simulink model "test_stepper_vector_space"  (R2020b)
settings: Solver=VariableStepAuto  StartTime=0.0  StopTime=10.0  RelTol=1e-3
undefined symbols (not defined in the file): const, controller, stepper
settings Model: Creator=Utente  LastModifiedBy=Utente

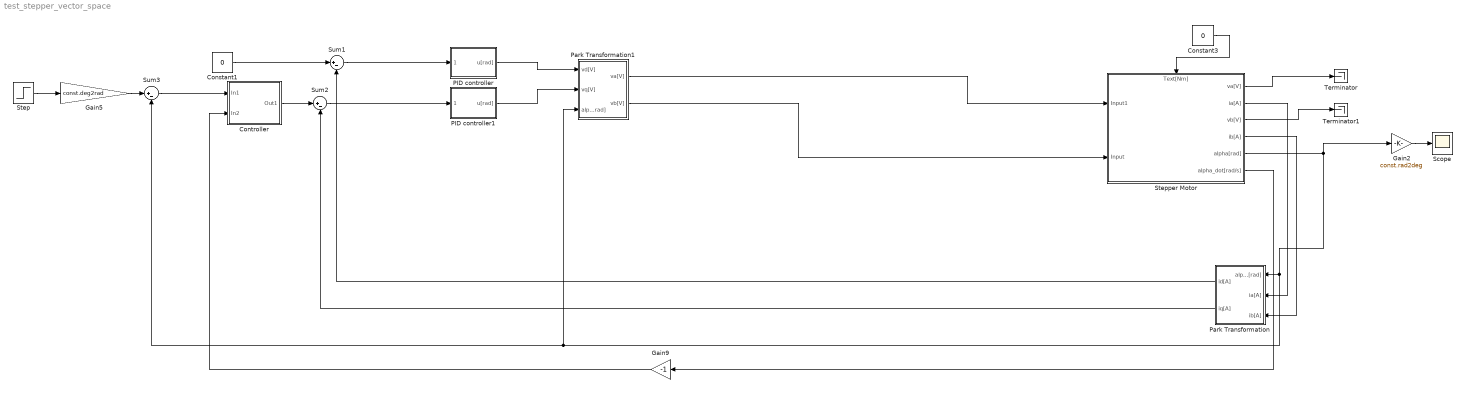
== system test_stepper_vector_space ==
  Constant1 : Constant  Value=0
  Constant3 : Constant  Value=0
  Controller : Subsystem
  Gain2 : Gain  Gain=const.rad2deg
  Gain5 : Gain  Gain=const.deg2rad
  Gain9 : Gain  Gain=-1
  PID controller : Subsystem
  PID controller1 : Subsystem
  Park Transformation : Subsystem
  Park Transformation1 : Subsystem
  Scope : Scope
  Step : Step  Time=0.1  After=30  SampleTime=0
  Stepper Motor : Subsystem
      settings: PortSchema="{\"entries\":[{\"content\":{\"sides\":[{\"content\":{\"connectorIds\":[\"In1\",\"In2\"]},\"type\":\"ConnectorPlacement.EquallySpacedRectSide\",\"uuid\":\"73295f7e-2188-4526-b3fe-31d6eab8afcb\"},{\"content\":{\"connectorIds\":[\"Out1\",\"Out2\",\"Out3\",\"Out4\",\"Out5\",\"Out6\"],\"side\":\"RIGHT\"},\"type\":\"ConnectorPlacement.EquallySpacedRectSide\",\"uuid\":\"77dcaa74-ce65-4a13-97c5-e825e2410182\"},{\"content\":{\"connectorIds\":[\"In3\"],\"side\":\"TOP\"},\"type\":\"ConnectorPlacement.EquallySpacedRectSide\",\"uuid\":\"bac6b674-d00a-4490-8f08-a2567c8e6873\"},{\"content\":{\"connectorIds\":[],\"side\":\"HIDDEN\"},\"type\":\"ConnectorPlacement.EquallySpacedRectSide\",\"uuid\":\"66c41dc0-366a-490c-a787-062f795e6cc7\"}]},\"type\":\"ConnectorPlacement.EquallySpacedConnector\",\"uuid\":\"3c22aa21-f88d-4b07-855c-a69922a8689b\"}],\"packageUris\":[\"http://schema.mathworks.com/mf0/Connector/R2020b\"],\"version\":\"1.0\"}"
  Sum1 : Sum  Inputs=|+-
  Sum2 : Sum  Inputs=|+-
  Sum3 : Sum  Inputs=|+-
  Terminator : Terminator
  Terminator1 : Terminator
  wires:
  Sum2/1 -> PID controller1/1(e[deg])
  Gain5/1 -> Sum3/1
  Sum1/1 -> PID controller/1(e[deg])
  Step/1 -> Gain5/1
  Constant3/1 -> Stepper Motor/3(Text[Nm])
  Park Transformation/2(iq[A]) -> Sum2/2
  Park Transformation/1(id[A]) -> Sum1/2
  Constant1/1 -> Sum1/1
  Stepper Motor/5(alpha[rad]) -> Gain2/1, Park Transformation1/3(alpha[rad]), Sum3/2, Park Transformation/1(alpha[rad])
  Stepper Motor/2(ia[A]) -> Park Transformation/2(ia[A])
  Stepper Motor/4(ib[A]) -> Park Transformation/3(ib[A])
  Stepper Motor/6(alpha_dot[rad/s]) -> Gain9/1
  Sum3/1 -> Controller/1(In1)
  Gain9/1 -> Controller/2(In2)
  Controller/1(Out1) -> Sum2/1
  PID controller/1(u[rad]) -> Park Transformation1/1(vd[V])
  PID controller1/1(u[rad]) -> Park Transformation1/2(vq[V])
  Gain2/1 -> Scope/1
  Stepper Motor/1(va[V]) -> Terminator/1
  Stepper Motor/3(vb[V]) -> Terminator1/1
  Park Transformation1/1(va[V]) -> Stepper Motor/1(Input1)
  Park Transformation1/2(vb[V]) -> Stepper Motor/2(Input)

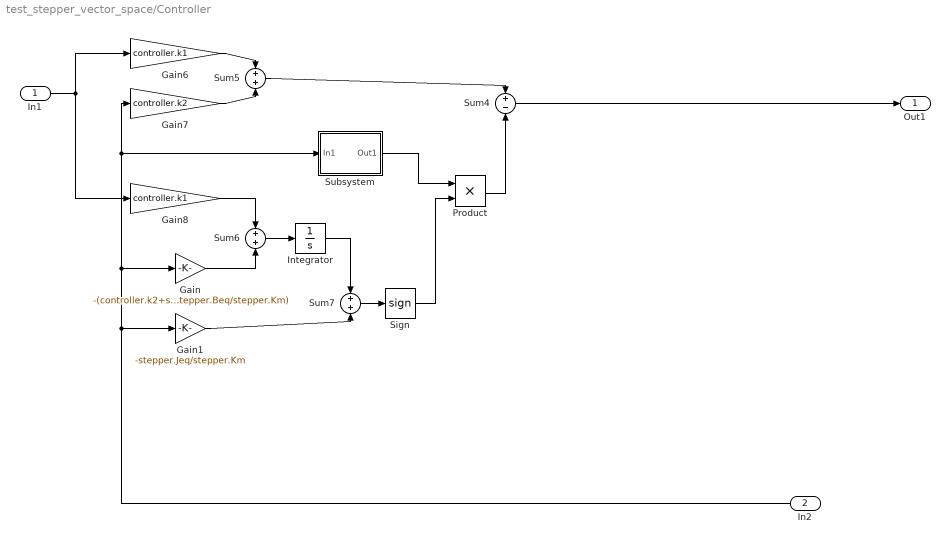
== system test_stepper_vector_space/Controller ==
  In1 : Inport
  In2 : Inport  Port=2
  Gain : Gain  Gain=-(controller.k2+stepper.Beq/stepper.Km)
  Gain1 : Gain  Gain=-stepper.Jeq/stepper.Km
  Gain6 : Gain  Gain=controller.k1
  Gain7 : Gain  Gain=controller.k2
  Gain8 : Gain  Gain=controller.k1
  Integrator : Integrator
  Product : Product
  Sign : Signum  ZeroCross=off
  Subsystem : Subsystem
  Sum4 : Sum  Inputs=+-
  Sum5 : Sum
  Sum6 : Sum
  Sum7 : Sum
  Out1 : Outport
  wires:
  In2/1 -> Subsystem/1(In1), Gain7/1, Gain/1, Gain1/1
  Sum5/1 -> Sum4/1
  Sum7/1 -> Sign/1
  Integrator/1 -> Sum7/1
  Gain1/1 -> Sum7/2
  Gain/1 -> Sum6/2
  Sum4/1 -> Out1/1
  In1/1 -> Gain6/1, Gain8/1
  Gain7/1 -> Sum5/2
  Gain6/1 -> Sum5/1
  Product/1 -> Sum4/2
  Sum6/1 -> Integrator/1
  Gain8/1 -> Sum6/1
  Subsystem/1(Out1) -> Product/1
  Sign/1 -> Product/2

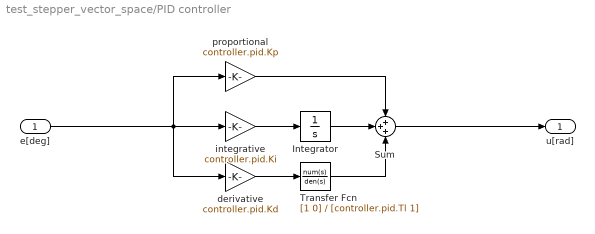
== system test_stepper_vector_space/PID controller ==
  e[deg] : Inport  Unit=deg
  Integrator : Integrator
  Sum : Sum  Inputs=+++
  Transfer Fcn : TransferFcn  Numerator=[1 0]  Denominator=[controller.pid.Tl 1]
  derivative : Gain  Gain=controller.pid.Kd
  integrative : Gain  Gain=controller.pid.Ki
  proportional : Gain  Gain=controller.pid.Kp
  u[rad] : Outport
  wires:
  Transfer Fcn/1 -> Sum/3
  e[deg]/1 -> derivative/1, proportional/1, integrative/1
  proportional/1 -> Sum/1
  integrative/1 -> Integrator/1
  Integrator/1 -> Sum/2
  Sum/1 -> u[rad]/1
  derivative/1 -> Transfer Fcn/1

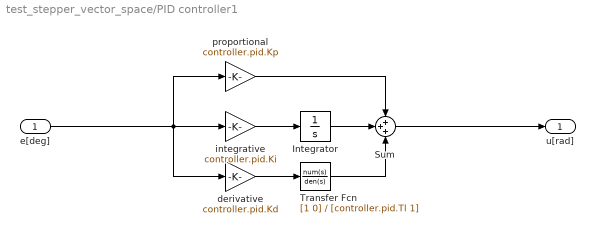
== system test_stepper_vector_space/PID controller1 ==
  e[deg] : Inport  Unit=deg
  Integrator : Integrator
  Sum : Sum  Inputs=+++
  Transfer Fcn : TransferFcn  Numerator=[1 0]  Denominator=[controller.pid.Tl 1]
  derivative : Gain  Gain=controller.pid.Kd
  integrative : Gain  Gain=controller.pid.Ki
  proportional : Gain  Gain=controller.pid.Kp
  u[rad] : Outport
  wires:
  Transfer Fcn/1 -> Sum/3
  e[deg]/1 -> derivative/1, proportional/1, integrative/1
  proportional/1 -> Sum/1
  integrative/1 -> Integrator/1
  Integrator/1 -> Sum/2
  Sum/1 -> u[rad]/1
  derivative/1 -> Transfer Fcn/1

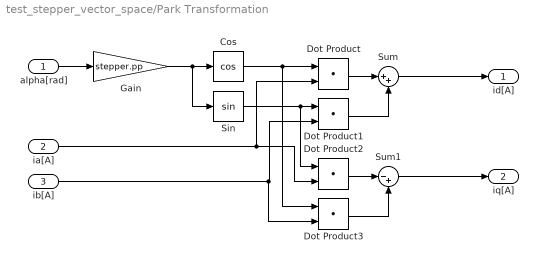
== system test_stepper_vector_space/Park Transformation ==
  alpha[rad] : Inport
  ia[A] : Inport  Port=2
  ib[A] : Inport  Port=3
  Cos : Trigonometry  Operator=cos
  Dot Product{,1..3} (4 alike) : DotProduct  InputSameDT=on  OutDataTypeStr=Inherit: Inherit via internal rule
  Gain : Gain  Gain=stepper.pp
  Sin : Trigonometry
  Sum : Sum  Inputs=|++
  Sum1 : Sum  Inputs=|-+
  id[A] : Outport
  iq[A] : Outport  Port=2
  wires:
  alpha[rad]/1 -> Gain/1
  Gain/1 -> Sin/1, Cos/1
  Cos/1 -> Dot Product3/1, Dot Product/1
  Dot Product/1 -> Sum/1
  ia[A]/1 -> Dot Product2/2, Dot Product/2
  Sin/1 -> Dot Product2/1, Dot Product1/1
  ib[A]/1 -> Dot Product3/2, Dot Product1/2
  Dot Product1/1 -> Sum/2
  Sum/1 -> id[A]/1
  Dot Product2/1 -> Sum1/1
  Dot Product3/1 -> Sum1/2
  Sum1/1 -> iq[A]/1

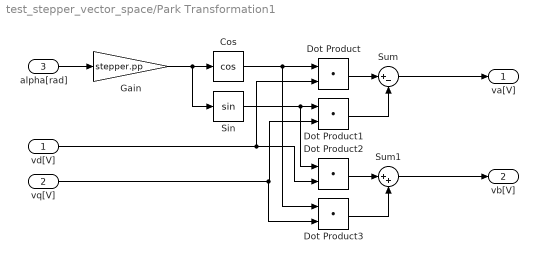
== system test_stepper_vector_space/Park Transformation1 ==
  vd[V] : Inport
  vq[V] : Inport  Port=2
  alpha[rad] : Inport  Port=3
  Cos : Trigonometry  Operator=cos
  Dot Product{,1..3} (4 alike) : DotProduct  InputSameDT=on  OutDataTypeStr=Inherit: Inherit via internal rule
  Gain : Gain  Gain=stepper.pp
  Sin : Trigonometry
  Sum : Sum  Inputs=|+-
  Sum1 : Sum  Inputs=|++
  va[V] : Outport
  vb[V] : Outport  Port=2
  wires:
  alpha[rad]/1 -> Gain/1
  Gain/1 -> Sin/1, Cos/1
  Cos/1 -> Dot Product3/1, Dot Product/1
  Dot Product/1 -> Sum/1
  vd[V]/1 -> Dot Product2/2, Dot Product/2
  Sin/1 -> Dot Product2/1, Dot Product1/1
  vq[V]/1 -> Dot Product3/2, Dot Product1/2
  Dot Product1/1 -> Sum/2
  Sum/1 -> va[V]/1
  Dot Product2/1 -> Sum1/1
  Dot Product3/1 -> Sum1/2
  Sum1/1 -> vb[V]/1

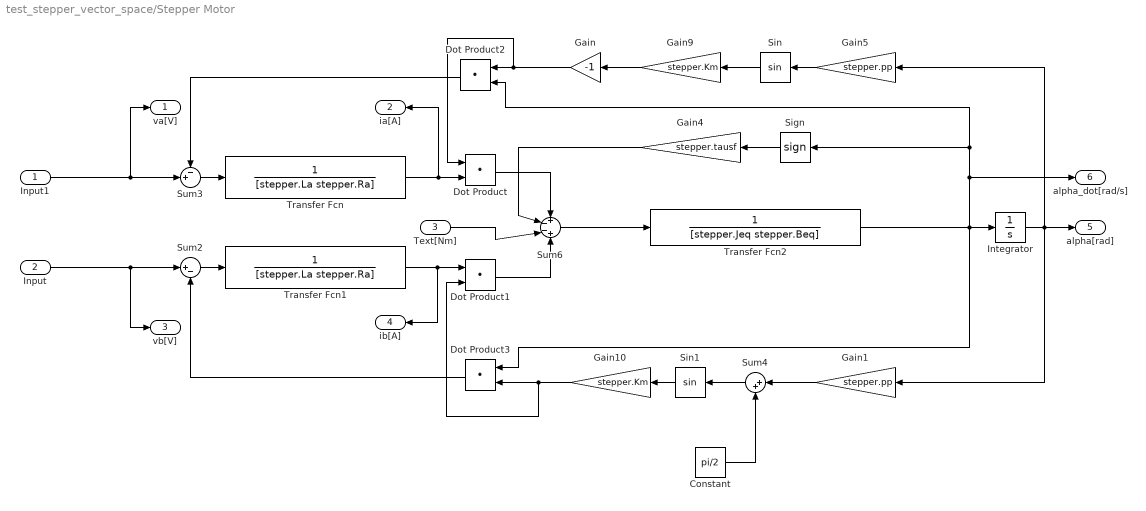
== system test_stepper_vector_space/Stepper Motor ==
  Input1 : Inport
  Input : Inport  Port=2
  Text[Nm] : Inport  Port=3
  Constant : Constant  Value=pi/2
  Dot Product{,1..3} (4 alike) : DotProduct  InputSameDT=on  OutDataTypeStr=Inherit: Inherit via internal rule
  Gain : Gain  Gain=-1
  Gain1 : Gain  Gain=stepper.pp
  Gain10 : Gain  Gain=stepper.Km
  Gain4 : Gain  Gain=stepper.tausf
  Gain5 : Gain  Gain=stepper.pp
  Gain9 : Gain  Gain=stepper.Km
  Integrator : Integrator
  Sign : Signum  ZeroCross=off
  Sin : Trigonometry
  Sin1 : Trigonometry
  Sum2 : Sum  Inputs=|+-
  Sum3 : Sum  Inputs=-+|
  Sum4 : Sum  Inputs=|++
  Sum6 : Sum  Inputs=+--+
  Transfer Fcn : TransferFcn  Denominator=[stepper.La stepper.Ra]
  Transfer Fcn1 : TransferFcn  Denominator=[stepper.La stepper.Ra]
  Transfer Fcn2 : TransferFcn  Denominator=[stepper.Jeq stepper.Beq]
  va[V] : Outport
  ia[A] : Outport  Port=2
  vb[V] : Outport  Port=3
  ib[A] : Outport  Port=4
  alpha[rad] : Outport  Port=5
  alpha_dot[rad/s] : Outport  Port=6
  wires:
  Input1/1 -> Sum3/2, va[V]/1
  Input/1 -> Sum2/1, vb[V]/1
  Sum3/1 -> Transfer Fcn/1
  Sum2/1 -> Transfer Fcn1/1
  Dot Product/1 -> Sum6/1
  Sum6/1 -> Transfer Fcn2/1
  Gain4/1 -> Sum6/2
  Transfer Fcn/1 -> Dot Product/2, ia[A]/1
  Transfer Fcn1/1 -> ib[A]/1, Dot Product1/1
  Gain5/1 -> Sin/1
  Integrator/1 -> Gain1/1, Gain5/1, alpha[rad]/1
  Transfer Fcn2/1 -> Dot Product3/1, Dot Product2/2, Sign/1, alpha_dot[rad/s]/1, Integrator/1
  Sin/1 -> Gain9/1
  Sin1/1 -> Gain10/1
  Dot Product3/1 -> Sum2/2
  Dot Product2/1 -> Sum3/1
  Gain10/1 -> Dot Product1/2, Dot Product3/2
  Sign/1 -> Gain4/1
  Gain9/1 -> Gain/1
  Dot Product1/1 -> Sum6/4
  Sum4/1 -> Sin1/1
  Gain1/1 -> Sum4/1
  Constant/1 -> Sum4/2
  Gain/1 -> Dot Product/1, Dot Product2/1
  Text[Nm]/1 -> Sum6/3

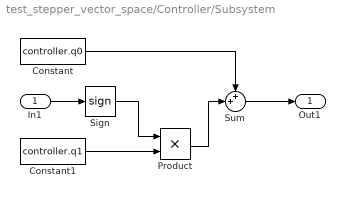
== system test_stepper_vector_space/Controller/Subsystem ==
  In1 : Inport
  Constant : Constant  Value=controller.q0
  Constant1 : Constant  Value=controller.q1
  Product : Product
  Sign : Signum  ZeroCross=off
  Sum : Sum  Inputs=++|
  Out1 : Outport
  wires:
  In1/1 -> Sign/1
  Sum/1 -> Out1/1
  Constant/1 -> Sum/1
  Constant1/1 -> Product/2
  Sign/1 -> Product/1
  Product/1 -> Sum/2
